simulink model "warplab_mimo_4x4"  (Simulink 6.5)
settings: Solver=ode45  StartTime=0.0  StopTime=20000  RelTol=1e-3
undefined symbols (not defined in the file): gcbh, xlBlockLoadCallback
libraries: xbsIndex_r4 x188
(part 2 of 17)

== system warplab_mimo_4x4/ System Generator ==
  2x System Clock : DiscretePulseGenerator  SampleTime=simulink_period
  Continuous Source : DiscretePulseGenerator  PulseType=Time based  Period=2*simulink_period  PulseWidth=50
  Terminator : Terminator
  Terminator1 : Terminator
  wires:
  2x System Clock/1 -> Terminator/1
  Continuous Source/1 -> Terminator1/1

== system warplab_mimo_4x4/CaptureDone ==
  In1 : Inport
  Inverter1 : S-Function  LoadFcn=xlBlockLoadCallback(gcbh);  FunctionName=sysgen  Parameters=ptable_  mask(Xilinx Inverter Block){infoedit=Bitwise logical negation (one's complement) operator., en_sgadvanced=, en=off, latency=0, dbl_ovrd_sgadvanced=, dbl_ovrd=off, xl_use_area_sgadvanced=, xl_use_area=off, xl_area=[0,0,0,0,0,0,0], has_advanced_control=0, sggui_pos=-1,-1,-1,-1, block_type=inv, block_version=8.2, sg_icon_stat=25,18,1,1,white,blue,0,1ab4a85f, sg_mask_display=|, sg_list_contents=, sg_blockgui_xml=}
      mask sg_mask_display=|
      | fprintf('','COMMENT: begin icon graphics');
      | patch([0 25 25 0 ],[0 0 18 18 ],[0.77 0.82 0.91]);
      | patch([8 5 9 5 8 13 14 15 20 16 12 9 13 9 12 16 20 15 14 13 8 ],[2 5 9 13 16 16 15 16 16 12 16 13 9 5 2 6 2 2 3 2 2 ],[0.98 0.96 0.92]);
      | plot([0 0 25 25 0 ],[0 18 18 0 0 ]);
      | fprintf('','COMMENT: end icon graphics');
      | fprintf('','COMMENT: begin icon text');
      | color('black');disp('not');
      | fprintf('','COMMENT: end icon text');
      mask prompts: infoedit ""; en_sgadvanced ""; en "Provide enable port"; dbl_ovrd_sgadvanced ""; dbl_ovrd "Override with doubles"; xl_use_area_sgadvanced ""; xl_use_area "Define FPGA area for resource estimation"; xl_area "FPGA area [slices, FFs, BRAMs, LUTs, IOBs, emb. mults, TBUFs]"; has_advanced_control ""; sggui_pos ""; block_type ""; block_version ""; sg_icon_stat ""; sg_mask_display ""; sg_list_contents ""; sg_blockgui_xml ""
      mask help: Bitwise logical negation (one's complement) operator.
      mask init: same as warplab_mimo_4x4/Inverter
      settings: CopyFcn=xlBlockMoveCallback(gcbh);  DeleteFcn=xlDestroyGui(gcbh);  ModelCloseFcn=xlDestroyGui(gcbh);  PreSaveFcn=xlBlockPreSaveCallback(gcbh);  PostSaveFcn=xlBlockPostSaveCallback(gcbh);  DestroyFcn=xlDestroyGui(gcbh);  OpenFcn=xlOpenGui(gcbh, 'inv_gui.xml', @xlmagicenablement, -1)  CloseFcn=xlDestroyGui(gcbh);  MoveFcn=xlBlockMoveCallback(gcbh);
      mask Help: eval('xlWeb(xlhtmldoclink(''Inverter''))');
      mask Display:
      | fprintf('','COMMENT: begin icon graphics');
      | patch([0 25 25 0 ],[0 0 18 18 ],[0.77 0.82 0.91]);
      | patch([8 5 9 5 8 13 14 15 20 16 12 9 13 9 12 16 20 15 14 13 8 ],[2 5 9 13 16 16 15 16 16 12 16 13 9 5 2 6 2 2 3 2 2 ],[0.98 0.96 0.92]);
      | plot([0 0 25 25 0 ],[0 18 18 0 0 ]);
      | fprintf('','COMMENT: end icon graphics');
      | fprintf('','COMMENT: begin icon text');
      | color('black');disp('not');
      | fprintf('','COMMENT: end icon text');
  zero3 : S-Function  LoadFcn=xlBlockLoadCallback(gcbh);  FunctionName=sysgen  Parameters=ptable_  mask(Xilinx Constant Block Block){arith_type_sgadvanced=, arith_type=Boolean, const=1, n_bits=1, bin_pt=0, explicit_period_sgadvanced=, explicit_period=off, period=1, dsp48_infoedit=The use of this block for DSP48 instructions is deprecated.  Please use the Opmode block., equ=P=C, opselect_sgadvanced=, opselect=C, inp2_sgadvanced=, inp2=PCIN>>17, opr_sgadvanced=, opr=+, inp1_sgadvanced=, inp1=P, carry_sgadvanced=, carry=CIN, dbl_ovrd_sgadvanced=, dbl_ovrd=off, has_advanced_control=0, sggui_pos=-1,-1,-1,-1, block_type=constant, block_version=VER_STRING_GOES_HERE, sg_icon_stat=20,18,0,1,white,blue,0,85613821, sg_mask_display=|, sg_list_contents=, sg_blockgui_xml=}
      mask sg_mask_display=|
      | fprintf('','COMMENT: begin icon graphics');
      | patch([0 55 55 0 ],[0 0 26 26 ],[0.77 0.82 0.91]);
      | patch([20 16 22 16 20 27 29 31 38 32 26 22 28 22 26 32 38 31 29 27 20 ],[3 7 13 19 23 23 21 23 23 17 23 19 13 7 3 9 3 3 5 3 3 ],[0.98 0.96 0.92]);
      | plot([0 0 55 55 0 ],[0 26 26 0 0 ]);
      | fprintf('','COMMENT: end icon graphics');
      | fprintf('','COMMENT: begin icon text');
      | color('black');port_label('output',1,'1');
      | fprintf('','COMMENT: end icon text');
      mask prompts: arith_type_sgadvanced ""; arith_type "Type"; const "Constant value"; n_bits "Number of bits"; bin_pt "Binary point"; explicit_period_sgadvanced ""; explicit_period "Sampled constant"; period "Sample period"; dsp48_infoedit ""; equ "DSP48 operation"; opselect_sgadvanced ""; opselect "Operation select"; inp2_sgadvanced ""; inp2 "Z mux"; opr_sgadvanced ""; opr "Operand"; inp1_sgadvanced ""; inp1 "YX muxes"; carry_sgadvanced ""; carry "Carry input"; dbl_ovrd_sgadvanced ""; dbl_ovrd "Override with doubles"; has_advanced_control ""; sggui_pos ""; block_type ""; block_version ""; sg_icon_stat ""; sg_mask_display ""; sg_list_contents ""; sg_blockgui_xml ""
      mask help: Xilinx Constant Block
      mask init:
      | try
      |   tmp_gcb = gcb;
      |   tmp_gcbh = gcbh;
      |   xlMungeMaskParams;
      |   block_config = 'sysgen_blockset:Constant_config';
      |   serialized_declarations = '{''arith_type''=>''Int'',''bin_pt''=>''Int'',''carry''=>''Int'',''const''=>''Double'',''dbl_ovrd''=>''Int'',''explicit_period''=>''Int'',''inp1''=>''Int'',''inp2''=>''Int'',''n_bits''=>''Int'',''opr''=>''Int'',''opselect''=>''Int'',''period''=>''Double''}';
      |   xlconstant_init();
      |   ptable_ = xlblockprep(get_param(tmp_gcb, 'MaskWSVariables'));
      | catch
      |   global dbgsysgen;
      |   if(~isempty(dbgsysgen) && dbgsysgen)
      |     e = regexprep(lasterr, '\n', '\nError: ');
      |     disp(['Error: While running MaskInit code on block ' tmp_gcb ': ' e]);
      |     error(e);
      |   end
      | end
      settings: CopyFcn=xlBlockMoveCallback(gcbh);  DeleteFcn=xlDestroyGui(gcbh);  ModelCloseFcn=xlDestroyGui(gcbh);  PreSaveFcn=xlBlockPreSaveCallback(gcbh);  PostSaveFcn=xlBlockPostSaveCallback(gcbh);  DestroyFcn=xlDestroyGui(gcbh);  OpenFcn=xlOpenGui(gcbh, 'constant_gui.xml', @constantenablement, @constantaction)  CloseFcn=xlDestroyGui(gcbh);  MoveFcn=xlBlockMoveCallback(gcbh);
      mask Help: eval('xlWeb(xlhtmldoclink(''Constant''))');
      mask StyleString: edit,popup(Boolean|Signed (2's comp)|Unsigned|DSP48 Instruction),edit,edit,edit,edit,checkbox,edit,edit,edit,edit,popup(C + A*B|PCIN + A*B|P + A*B|A * B|C + A:B|C - A:B|C|Custom),edit,popup(0|PCIN|P|C|PCIN>>17|P>>17),edit,popup(+|-),edit,popup(0|P|A:B|A*B|C|P+C|A:B+C),edit,popup(0|1|CIN|~SIGN(P or PCIN)|~SIGN(A*B or A:B)|~SIGND(A*B or A:B)),edit,checkbox,edit,edit,edit,edit,edit,edit,edit,edit
      mask Display:
      | fprintf('','COMMENT: begin icon graphics');
      | patch([0 55 55 0 ],[0 0 26 26 ],[0.77 0.82 0.91]);
      | patch([20 16 22 16 20 27 29 31 38 32 26 22 28 22 26 32 38 31 29 27 20 ],[3 7 13 19 23 23 21 23 23 17 23 19 13 7 3 9 3 3 5 3 3 ],[0.98 0.96 0.92]);
      | plot([0 0 55 55 0 ],[0 26 26 0 0 ]);
      | fprintf('','COMMENT: end icon graphics');
      | fprintf('','COMMENT: begin icon text');
      | color('black');port_label('output',1,'1');
      | fprintf('','COMMENT: end icon text');
  Out1_To_Register : Outport
  tag scope: en_out_13=global, out_13=global
  wires:
  In1/1 -> Inverter1/1
  Inverter1/1 -> [out_13]
  zero3/1 -> [en_out_13]

== system warplab_mimo_4x4/Mem_Control ==
  Start : Inport
  DoneReading : Inport  Port=2
  CaptOffset : Inport  Port=3
  AddSub1 : S-Function  LoadFcn=xlBlockLoadCallback(gcbh);  FunctionName=sysgen  Parameters=ptable_  mask(Xilinx Adder/Subtractor Block){mode_sgadvanced=, mode=Subtraction, use_carryin_sgadvanced=, use_carryin=off, use_carryout_sgadvanced=, use_carryout=off, en_sgadvanced=, en=off, latency=0, precision_sgadvanced=, precision=User Defined, arith_type_sgadvanced=, arith_type=Unsigned, n_bits=14, bin_pt=0, quantization_sgadvanced=, quantization=Truncate, overflow_sgadvanced=, overflow=Wrap, dbl_ovrd_sgadvanced=, dbl_ovrd=off, use_behavioral_HDL_sgadvanced=, use_behavioral_HDL=off, pipelined_sgadvanced=, pipelined=off, use_rpm_sgadvanced=, use_rpm=on, xl_use_area_sgadvanced=, xl_use_area=off, xl_area=[0,0,0,0,0,0,0], has_advanced_control=0, sggui_pos=-1,-1,-1,-1, block_type=addsub, block_version=8.2, sg_icon_stat=45,38,2,1,white,blue,0,f28631c4, sg_mask_display=|, sg_list_contents=, sg_blockgui_xml=}
      mask sg_mask_display=|
      | fprintf('','COMMENT: begin icon graphics');
      | patch([0 45 45 0 ],[0 0 38 38 ],[0.77 0.82 0.91]);
      | patch([12 6 15 6 12 22 25 28 39 31 23 17 26 17 23 31 39 28 25 22 12 ],[4 10 19 28 34 34 31 34 34 26 34 28 19 10 4 12 4 4 7 4 4 ],[0.98 0.96 0.92]);
      | plot([0 0 45 45 0 ],[0 38 38 0 0 ]);
      | fprintf('','COMMENT: end icon graphics');
      | fprintf('','COMMENT: begin icon text');
      | color('black');port_label('input',1,'a');
      | color('black');port_label('input',2,'b');
      | color('black');port_label('output',1,'\bf{a - b}','texmode','on');
      | fprintf('','COMMENT: end icon text');
      mask prompts: mode_sgadvanced ""; mode "Operation"; use_carryin_sgadvanced ""; use_carryin "Provide carry-in port"; use_carryout_sgadvanced ""; use_carryout "Provide carry-out port"; en_sgadvanced ""; en "Provide enable port"; precision_sgadvanced ""; arith_type_sgadvanced ""; arith_type "Output type"; n_bits "Number of bits"; bin_pt "Binary point"; quantization_sgadvanced ""; overflow_sgadvanced ""; dbl_ovrd_sgadvanced ""; dbl_ovrd "Override with doubles"; use_behavioral_HDL_sgadvanced ""; use_behavioral_HDL "Use behavioral HDL (otherwise use core)"; pipelined_sgadvanced ""; pipelined "Pipeline for maximum performance"; use_rpm_sgadvanced ""; use_rpm "Use core placement information"; xl_use_area_sgadvanced ""; xl_use_area "Define FPGA area for resource estimation"; xl_area "FPGA area [slices, FFs, BRAMs, LUTs, IOBs, emb. mults, TBUFs]"; has_advanced_control ""; sggui_pos ""; block_type ""; block_version ""; sg_icon_stat ""; sg_mask_display ""; sg_list_contents ""; sg_blockgui_xml ""
      mask help: Xilinx Adder/Subtractor
      mask init:
      | try
      |   tmp_gcb = gcb;
      |   tmp_gcbh = gcbh;
      |   xlMungeMaskParams;
      |   block_config = 'sysgen_blockset:Addsub_config';
      |   serialized_declarations = '{''arith_type''=>''Int'',''bin_pt''=>''Int'',''en''=>''Int'',''latency''=>''Int'',''mode''=>''Int'',''n_bits''=>''Int'',''overflow''=>''Int'',''pipelined''=>''Int'',''precision''=>''Int'',''quantization''=>''Int'',''rst''=>''Int'',''use_behavioral_HDL''=>''Int'',''use_carryin''=>''Int'',''use_carryout''=>''Int'',''use_rpm''=>''Int''}';
      |   ptable_ = xlblockprep(get_param(tmp_gcb, 'MaskWSVariables'));
      | catch
      |   global dbgsysgen;
      |   if(~isempty(dbgsysgen) && dbgsysgen)
      |     e = regexprep(lasterr, '\n', '\nError: ');
      |     disp(['Error: While running MaskInit code on block ' tmp_gcb ': ' e]);
      |     error(e);
      |   end
      | end
      settings: CopyFcn=xlBlockMoveCallback(gcbh);  DeleteFcn=xlDestroyGui(gcbh);  ModelCloseFcn=xlDestroyGui(gcbh);  PreSaveFcn=xlBlockPreSaveCallback(gcbh);  PostSaveFcn=xlBlockPostSaveCallback(gcbh);  DestroyFcn=xlDestroyGui(gcbh);  OpenFcn=xlOpenGui(gcbh, 'addsub_gui.xml', @addsubenablement, -1)  CloseFcn=xlDestroyGui(gcbh);  MoveFcn=xlBlockMoveCallback(gcbh);
      mask Help: eval('xlWeb(xlhtmldoclink(''AddSub''))');
      mask StyleString: edit,popup(Addition|Subtraction|Addition or Subtraction),edit,checkbox,edit,checkbox,edit,checkbox,edit,edit,popup(Full|User Defined),edit,popup(Signed  (2's comp)|Unsigned),edit,edit,edit,popup(Truncate|Round  (unbiased: +/- Inf)),edit,popup(Wrap|Saturate|Flag as error),edit,checkbox,edit,checkbox,edit,checkbox,edit,checkbox,edit,checkbox,edit,edit,edit,edit,edit,edit,edit,edit,edit
      mask Display:
      | fprintf('','COMMENT: begin icon graphics');
      | patch([0 45 45 0 ],[0 0 38 38 ],[0.77 0.82 0.91]);
      | patch([12 6 15 6 12 22 25 28 39 31 23 17 26 17 23 31 39 28 25 22 12 ],[4 10 19 28 34 34 31 34 34 26 34 28 19 10 4 12 4 4 7 4 4 ],[0.98 0.96 0.92]);
      | plot([0 0 45 45 0 ],[0 38 38 0 0 ]);
      | fprintf('','COMMENT: end icon graphics');
      | fprintf('','COMMENT: begin icon text');
      | color('black');port_label('input',1,'a');
      | color('black');port_label('input',2,'b');
      | color('black');port_label('output',1,'\bf{a - b}','texmode','on');
      | fprintf('','COMMENT: end icon text');
  Convert1 : S-Function  LoadFcn=xlBlockLoadCallback(gcbh);  FunctionName=sysgen  Parameters=ptable_  mask(Xilinx Type Converter Block){infoedit=Hardware notes: rounding and saturating require hardware resources; truncating and wrapping do not., arith_type_sgadvanced=, arith_type=Boolean, n_bits=16, bin_pt=14, quantization_sgadvanced=, quantization=Truncate, overflow_sgadvanced=, overflow=Wrap, latency=0, dbl_ovrd_sgadvanced=, dbl_ovrd=off, pipeline_sgadvanced=, pipeline=off, xl_use_area_sgadvanced=, xl_use_area=off, xl_area=[0,0,0,0,0,0,0], has_advanced_control=0, sggui_pos=20,20,374,375, block_type=convert, block_version=8.2, sg_icon_stat=35,18,1,1,white,blue,0,0eb6e735, sg_mask_display=|, sg_list_contents=, sg_blockgui_xml=}
      mask sg_mask_display=|
      | fprintf('','COMMENT: begin icon graphics');
      | patch([0 35 35 0 ],[0 0 18 18 ],[0.77 0.82 0.91]);
      | patch([13 10 14 10 13 18 19 20 25 21 17 14 18 14 17 21 25 20 19 18 13 ],[2 5 9 13 16 16 15 16 16 12 16 13 9 5 2 6 2 2 3 2 2 ],[0.98 0.96 0.92]);
      | plot([0 0 35 35 0 ],[0 18 18 0 0 ]);
      | fprintf('','COMMENT: end icon graphics');
      | fprintf('','COMMENT: begin icon text');
      | color('black');port_label('output',1,'cast');
      | fprintf('','COMMENT: end icon text');
      mask prompts: infoedit ""; arith_type_sgadvanced ""; arith_type "Type"; n_bits "Number of bits"; bin_pt "Binary point"; quantization_sgadvanced ""; overflow_sgadvanced ""; dbl_ovrd_sgadvanced ""; dbl_ovrd "Override with doubles"; pipeline_sgadvanced ""; pipeline "Pipeline for maximum performance"; xl_use_area_sgadvanced ""; xl_use_area "Define FPGA area for resource estimation"; xl_area "FPGA area [slices, FFs, BRAMs, LUTs, IOBs, emb. mults, TBUFs]"; has_advanced_control ""; sggui_pos ""; block_type ""; block_version ""; sg_icon_stat ""; sg_mask_display ""; sg_list_contents ""; sg_blockgui_xml ""
      mask help: Hardware notes: rounding and saturating require hardware resources; truncating and wrapping do not.
      mask init:
      | try
      |   tmp_gcb = gcb;
      |   tmp_gcbh = gcbh;
      |   xlMungeMaskParams;
      |   block_config = 'sysgen_blockset:Convert_config';
      |   serialized_declarations = '{''arith_type''=>''Int'',''bin_pt''=>''Int'',''latency''=>''Int'',''n_bits''=>''Int'',''overflow''=>''Int'',''pipeline''=>''Int'',''quantization''=>''Int'',''sim_engine''=>''Int'',''sysgen_root''=>''String''}';
      |   xlconvert_init();
      |   ptable_ = xlblockprep(get_param(tmp_gcb, 'MaskWSVariables'));
      | catch
      |   global dbgsysgen;
      |   if(~isempty(dbgsysgen) && dbgsysgen)
      |     e = regexprep(lasterr, '\n', '\nError: ');
      |     disp(['Error: While running MaskInit code on block ' tmp_gcb ': ' e]);
      |     error(e);
      |   end
      | end
      settings: CopyFcn=xlBlockMoveCallback(gcbh);  DeleteFcn=xlDestroyGui(gcbh);  ModelCloseFcn=xlDestroyGui(gcbh);  PreSaveFcn=xlBlockPreSaveCallback(gcbh);  PostSaveFcn=xlBlockPostSaveCallback(gcbh);  DestroyFcn=xlDestroyGui(gcbh);  OpenFcn=xlOpenGui(gcbh, 'convert_gui.xml', @convertenablement, -1)  CloseFcn=xlDestroyGui(gcbh);  MoveFcn=xlBlockMoveCallback(gcbh);
      mask Help: eval('xlWeb(xlhtmldoclink(''Convert''))');
      mask StyleString: edit,edit,popup(Boolean|Signed  (2's comp)|Unsigned),edit,edit,edit,popup(Truncate|Round  (unbiased: +/- Inf)|Round  (unbiased: Even Values)),edit,popup(Wrap|Saturate|Flag as error),edit,edit,checkbox,edit,checkbox,edit,checkbox,edit,edit,edit,edit,edit,edit,edit,edit,edit
      mask Display:
      | fprintf('','COMMENT: begin icon graphics');
      | patch([0 35 35 0 ],[0 0 18 18 ],[0.77 0.82 0.91]);
      | patch([13 10 14 10 13 18 19 20 25 21 17 14 18 14 17 21 25 20 19 18 13 ],[2 5 9 13 16 16 15 16 16 12 16 13 9 5 2 6 2 2 3 2 2 ],[0.98 0.96 0.92]);
      | plot([0 0 35 35 0 ],[0 18 18 0 0 ]);
      | fprintf('','COMMENT: end icon graphics');
      | fprintf('','COMMENT: begin icon text');
      | color('black');port_label('output',1,'cast');
      | fprintf('','COMMENT: end icon text');
  Delay : S-Function  LoadFcn=xlBlockLoadCallback(gcbh);  FunctionName=sysgen  Parameters=ptable_  mask(Xilinx Delay Block){infoedit=Hardware notes: A delay line is a chain, each link of which is an SRL16 followed by a flip-flop. If register retiming is enabled, the delay line is a chain of flip-flops., en_sgadvanced=, en=off, latency=1, dbl_ovrd_sgadvanced=, dbl_ovrd=off, reg_retiming_sgadvanced=, reg_retiming=off, xl_use_area_sgadvanced=, xl_use_area=off, xl_area=[0,0,0,0,0,0,0], has_advanced_control=0, sggui_pos=-1,-1,-1,-1, block_type=delay, block_version=8.2, sg_icon_stat=30,30,1,1,white,blue,0,fc531c0e, sg_mask_display=|, sg_list_contents=, sg_blockgui_xml=}
      mask sg_mask_display=|
      | fprintf('','COMMENT: begin icon graphics');
      | patch([0 30 30 0 ],[0 0 30 30 ],[0.77 0.82 0.91]);
      | patch([7 2 9 2 7 15 17 19 27 20 14 9 15 9 14 20 27 19 17 15 7 ],[3 8 15 22 27 27 25 27 27 20 26 21 15 9 4 10 3 3 5 3 3 ],[0.98 0.96 0.92]);
      | plot([0 0 30 30 0 ],[0 30 30 0 0 ]);
      | fprintf('','COMMENT: end icon graphics');
      | fprintf('','COMMENT: begin icon text');
      | color('black');disp('z^{-1}','texmode','on');
      | fprintf('','COMMENT: end icon text');
      mask prompts: infoedit ""; en_sgadvanced ""; en "Provide enable port"; dbl_ovrd_sgadvanced ""; dbl_ovrd "Override with doubles"; reg_retiming_sgadvanced ""; reg_retiming "Implement using behavioral HDL."; xl_use_area_sgadvanced ""; xl_use_area "Define FPGA area for resource estimation"; xl_area "FPGA area [slices, FFs, BRAMs, LUTs, IOBs, emb. mults, TBUFs]"; has_advanced_control ""; sggui_pos ""; block_type ""; block_version ""; sg_icon_stat ""; sg_mask_display ""; sg_list_contents ""; sg_blockgui_xml ""
      mask help: Hardware notes: A delay line is a chain, each link of which is an SRL16 followed by a flip-flop.
      mask init:
      | try
      |   tmp_gcb = gcb;
      |   tmp_gcbh = gcbh;
      |   xlMungeMaskParams;
      |   block_config = 'sysgen_blockset:Delay_config';
      |   serialized_declarations = '{''dbl_ovrd''=>''Int'',''en''=>''Int'',''latency''=>''Int'',''reg_retiming''=>''Int''}';
      |   ptable_ = xlblockprep(get_param(tmp_gcb, 'MaskWSVariables'));
      | catch
      |   global dbgsysgen;
      |   if(~isempty(dbgsysgen) && dbgsysgen)
      |     e = regexprep(lasterr, '\n', '\nError: ');
      |     disp(['Error: While running MaskInit code on block ' tmp_gcb ': ' e]);
      |     error(e);
      |   end
      | end
      settings: CopyFcn=xlBlockMoveCallback(gcbh);  DeleteFcn=xlDestroyGui(gcbh);  ModelCloseFcn=xlDestroyGui(gcbh);  PreSaveFcn=xlBlockPreSaveCallback(gcbh);  PostSaveFcn=xlBlockPostSaveCallback(gcbh);  DestroyFcn=xlDestroyGui(gcbh);  OpenFcn=xlOpenGui(gcbh, 'delay_gui.xml', @xlmagicenablement, -1)  CloseFcn=xlDestroyGui(gcbh);  MoveFcn=xlBlockMoveCallback(gcbh);
      mask Help: eval('xlWeb(xlhtmldoclink(''Delay''))');
      mask Display:
      | fprintf('','COMMENT: begin icon graphics');
      | patch([0 30 30 0 ],[0 0 30 30 ],[0.77 0.82 0.91]);
      | patch([7 2 9 2 7 15 17 19 27 20 14 9 15 9 14 20 27 19 17 15 7 ],[3 8 15 22 27 27 25 27 27 20 26 21 15 9 4 10 3 3 5 3 3 ],[0.98 0.96 0.92]);
      | plot([0 0 30 30 0 ],[0 30 30 0 0 ]);
      | fprintf('','COMMENT: end icon graphics');
      | fprintf('','COMMENT: begin icon text');
      | color('black');disp('z^{-1}','texmode','on');
      | fprintf('','COMMENT: end icon text');
  Logical : S-Function  LoadFcn=xlBlockLoadCallback(gcbh);  FunctionName=sysgen  Parameters=ptable_  mask(Xilinx Logical Block Block){logical_function_sgadvanced=, logical_function=AND, inputs=2, en_sgadvanced=, en=off, latency=0, precision_sgadvanced=, precision=Full, arith_type_sgadvanced=, arith_type=Unsigned, n_bits=16, bin_pt=0, align_bp_sgadvanced=, align_bp=on, dbl_ovrd_sgadvanced=, dbl_ovrd=off, xl_use_area_sgadvanced=, xl_use_area=off, xl_area=[0,0,0,0,0,0,0], overflow=, quantization=, has_advanced_control=0, sggui_pos=-1,-1,-1,-1, block_type=logical, block_version=8.2, sg_icon_stat=35,42,2,1,white,blue,0,087b5522, sg_mask_display=|, sg_list_contents=, sg_blockgui_xml=}
      mask sg_mask_display=|
      | fprintf('','COMMENT: begin icon graphics');
      | patch([0 35 35 0 ],[0 0 42 42 ],[0.77 0.82 0.91]);
      | patch([8 2 10 2 8 17 20 23 33 25 18 13 21 13 18 25 33 23 20 17 8 ],[7 13 21 29 35 35 32 35 35 27 34 29 21 13 8 15 7 7 10 7 7 ],[0.98 0.96 0.92]);
      | plot([0 0 35 35 0 ],[0 42 42 0 0 ]);
      | fprintf('','COMMENT: end icon graphics');
      | fprintf('','COMMENT: begin icon text');
      | color('black');disp('\newlineand\newlinez^{-0}','texmode','on');
      | fprintf('','COMMENT: end icon text');
      mask prompts: logical_function_sgadvanced ""; logical_function "Logical function"; inputs "Number of inputs"; en_sgadvanced ""; en "Provide enable port"; precision_sgadvanced ""; arith_type_sgadvanced ""; arith_type "Output Type"; n_bits "Number of bits"; bin_pt "Binary point"; align_bp_sgadvanced ""; align_bp "Align binary point"; dbl_ovrd_sgadvanced ""; dbl_ovrd "Override with doubles"; xl_use_area_sgadvanced ""; xl_use_area "Define FPGA area for resource estimation"; xl_area "FPGA area [slices, FFs, BRAMs, LUTs, IOBs, emb. mults, TBUFs]"; overflow ""; quantization ""; has_advanced_control ""; sggui_pos ""; block_type ""; block_version ""; sg_icon_stat ""; sg_mask_display ""; sg_list_contents ""; sg_blockgui_xml ""
      mask help: Xilinx Logical Block
      mask init: same as warplab_mimo_4x4/Logical
      settings: CopyFcn=xlBlockMoveCallback(gcbh);  DeleteFcn=xlDestroyGui(gcbh);  ModelCloseFcn=xlDestroyGui(gcbh);  PreSaveFcn=xlBlockPreSaveCallback(gcbh);  PostSaveFcn=xlBlockPostSaveCallback(gcbh);  DestroyFcn=xlDestroyGui(gcbh);  OpenFcn=xlOpenGui(gcbh, 'logical_gui.xml', @logicalenablement, -1)  CloseFcn=xlDestroyGui(gcbh);  MoveFcn=xlBlockMoveCallback(gcbh);
      mask Help: eval('xlWeb(xlhtmldoclink(''Logical''))');
      mask StyleString: edit,popup(AND|NAND|OR|NOR|XOR|XNOR),edit,edit,checkbox,edit,edit,popup(Full|User Defined),edit,popup(Signed  (2's comp)|Unsigned),edit,edit,edit,checkbox,edit,checkbox,edit,checkbox,edit,edit,edit,edit,edit,edit,edit,edit,edit,edit,edit
      mask Display:
      | fprintf('','COMMENT: begin icon graphics');
      | patch([0 35 35 0 ],[0 0 42 42 ],[0.77 0.82 0.91]);
      | patch([8 2 10 2 8 17 20 23 33 25 18 13 21 13 18 25 33 23 20 17 8 ],[7 13 21 29 35 35 32 35 35 27 34 29 21 13 8 15 7 7 10 7 7 ],[0.98 0.96 0.92]);
      | plot([0 0 35 35 0 ],[0 42 42 0 0 ]);
      | fprintf('','COMMENT: end icon graphics');
      | fprintf('','COMMENT: begin icon text');
      | color('black');disp('\newlineand\newlinez^{-0}','texmode','on');
      | fprintf('','COMMENT: end icon text');
  Logical2 : S-Function  LoadFcn=xlBlockLoadCallback(gcbh);  FunctionName=sysgen  Parameters=ptable_  mask(Xilinx Logical Block Block){logical_function_sgadvanced=, logical_function=AND, inputs=2, en_sgadvanced=, en=off, latency=0, precision_sgadvanced=, precision=Full, arith_type_sgadvanced=, arith_type=Unsigned, n_bits=16, bin_pt=0, align_bp_sgadvanced=, align_bp=on, dbl_ovrd_sgadvanced=, dbl_ovrd=off, xl_use_area_sgadvanced=, xl_use_area=off, xl_area=[0,0,0,0,0,0,0], overflow=, quantization=, has_advanced_control=0, sggui_pos=-1,-1,-1,-1, block_type=logical, block_version=8.2, sg_icon_stat=35,42,2,1,white,blue,0,087b5522, sg_mask_display=|, sg_list_contents=, sg_blockgui_xml=}
      mask sg_mask_display=|
      | fprintf('','COMMENT: begin icon graphics');
      | patch([0 35 35 0 ],[0 0 42 42 ],[0.77 0.82 0.91]);
      | patch([8 2 10 2 8 17 20 23 33 25 18 13 21 13 18 25 33 23 20 17 8 ],[7 13 21 29 35 35 32 35 35 27 34 29 21 13 8 15 7 7 10 7 7 ],[0.98 0.96 0.92]);
      | plot([0 0 35 35 0 ],[0 42 42 0 0 ]);
      | fprintf('','COMMENT: end icon graphics');
      | fprintf('','COMMENT: begin icon text');
      | color('black');disp('\newlineand\newlinez^{-0}','texmode','on');
      | fprintf('','COMMENT: end icon text');
      mask prompts: logical_function_sgadvanced ""; logical_function "Logical function"; inputs "Number of inputs"; en_sgadvanced ""; en "Provide enable port"; precision_sgadvanced ""; arith_type_sgadvanced ""; arith_type "Output Type"; n_bits "Number of bits"; bin_pt "Binary point"; align_bp_sgadvanced ""; align_bp "Align binary point"; dbl_ovrd_sgadvanced ""; dbl_ovrd "Override with doubles"; xl_use_area_sgadvanced ""; xl_use_area "Define FPGA area for resource estimation"; xl_area "FPGA area [slices, FFs, BRAMs, LUTs, IOBs, emb. mults, TBUFs]"; overflow ""; quantization ""; has_advanced_control ""; sggui_pos ""; block_type ""; block_version ""; sg_icon_stat ""; sg_mask_display ""; sg_list_contents ""; sg_blockgui_xml ""
      mask help: Xilinx Logical Block
      mask init: same as warplab_mimo_4x4/Logical
      settings: CopyFcn=xlBlockMoveCallback(gcbh);  DeleteFcn=xlDestroyGui(gcbh);  ModelCloseFcn=xlDestroyGui(gcbh);  PreSaveFcn=xlBlockPreSaveCallback(gcbh);  PostSaveFcn=xlBlockPostSaveCallback(gcbh);  DestroyFcn=xlDestroyGui(gcbh);  OpenFcn=xlOpenGui(gcbh, 'logical_gui.xml', @logicalenablement, -1)  CloseFcn=xlDestroyGui(gcbh);  MoveFcn=xlBlockMoveCallback(gcbh);
      mask Help: eval('xlWeb(xlhtmldoclink(''Logical''))');
      mask StyleString: edit,popup(AND|NAND|OR|NOR|XOR|XNOR),edit,edit,checkbox,edit,edit,popup(Full|User Defined),edit,popup(Signed  (2's comp)|Unsigned),edit,edit,edit,checkbox,edit,checkbox,edit,checkbox,edit,edit,edit,edit,edit,edit,edit,edit,edit,edit,edit
      mask Display:
      | fprintf('','COMMENT: begin icon graphics');
      | patch([0 35 35 0 ],[0 0 42 42 ],[0.77 0.82 0.91]);
      | patch([8 2 10 2 8 17 20 23 33 25 18 13 21 13 18 25 33 23 20 17 8 ],[7 13 21 29 35 35 32 35 35 27 34 29 21 13 8 15 7 7 10 7 7 ],[0.98 0.96 0.92]);
      | plot([0 0 35 35 0 ],[0 42 42 0 0 ]);
      | fprintf('','COMMENT: end icon graphics');
      | fprintf('','COMMENT: begin icon text');
      | color('black');disp('\newlineand\newlinez^{-0}','texmode','on');
      | fprintf('','COMMENT: end icon text');
  Register : S-Function  LoadFcn=xlBlockLoadCallback(gcbh);  FunctionName=sysgen  Parameters=ptable_  mask(Xilinx Register Block){init=0, rst_sgadvanced=, rst=off, en_sgadvanced=, en=on, dbl_ovrd_sgadvanced=, dbl_ovrd=off, xl_use_area_sgadvanced=, xl_use_area=off, xl_area=[0,0,0,0,0,0,0], has_advanced_control=0, sggui_pos=-1,-1,-1,-1, block_type=register, block_version=8.2, sg_icon_stat=50,40,2,1,white,blue,0,cc3303a0, sg_mask_display=|, sg_list_contents=, sg_blockgui_xml=}
      mask sg_mask_display=|
      | fprintf('','COMMENT: begin icon graphics');
      | patch([0 50 50 0 ],[0 0 40 40 ],[0.77 0.82 0.91]);
      | patch([15 8 17 8 15 26 29 32 43 34 25 19 29 19 25 34 43 32 29 26 15 ],[4 11 20 29 36 36 33 36 36 27 36 30 20 10 4 13 4 4 7 4 4 ],[0.98 0.96 0.92]);
      | plot([0 0 50 50 0 ],[0 40 40 0 0 ]);
      | fprintf('','COMMENT: end icon graphics');
      | fprintf('','COMMENT: begin icon text');
      | color('black');port_label('input',1,'d');
      | color('black');port_label('input',2,'en');
      | color('black');port_label('output',1,'q');
      | color('black');disp('\bf{z^{-1}}','texmode','on');
      | fprintf('','COMMENT: end icon text');
      mask prompts: init "Initial value"; rst_sgadvanced ""; rst "Provide synchronous reset port"; en_sgadvanced ""; en "Provide enable port"; dbl_ovrd_sgadvanced ""; dbl_ovrd "Override with doubles"; xl_use_area_sgadvanced ""; xl_use_area "Define FPGA area for resource estimation"; xl_area "FPGA area [slices, FFs, BRAMs, LUTs, IOBs, emb. mults, TBUFs]"; has_advanced_control ""; sggui_pos ""; block_type ""; block_version ""; sg_icon_stat ""; sg_mask_display ""; sg_list_contents ""; sg_blockgui_xml ""
      mask help: Xilinx Register
      mask init:
      | try
      |   tmp_gcb = gcb;
      |   tmp_gcbh = gcbh;
      |   xlMungeMaskParams;
      |   block_config = 'sysgen_blockset:Register_config';
      |   serialized_declarations = '{''dbl_ovrd''=>''Int'',''en''=>''Int'',''init''=>''Double'',''rst''=>''Int''}';
      |   xlregister_init();
      |   ptable_ = xlblockprep(get_param(tmp_gcb, 'MaskWSVariables'));
      | catch
      |   global dbgsysgen;
      |   if(~isempty(dbgsysgen) && dbgsysgen)
      |     e = regexprep(lasterr, '\n', '\nError: ');
      |     disp(['Error: While running MaskInit code on block ' tmp_gcb ': ' e]);
      |     error(e);
      |   end
      | end
      settings: CopyFcn=xlBlockMoveCallback(gcbh);  DeleteFcn=xlDestroyGui(gcbh);  ModelCloseFcn=xlDestroyGui(gcbh);  PreSaveFcn=xlBlockPreSaveCallback(gcbh);  PostSaveFcn=xlBlockPostSaveCallback(gcbh);  DestroyFcn=xlDestroyGui(gcbh);  OpenFcn=xlOpenGui(gcbh, 'register_gui.xml', @xlmagicenablement, -1)  CloseFcn=xlDestroyGui(gcbh);  MoveFcn=xlBlockMoveCallback(gcbh);
      mask Help: eval('xlWeb(xlhtmldoclink(''Register''))');
      mask Display:
      | fprintf('','COMMENT: begin icon graphics');
      | patch([0 50 50 0 ],[0 0 40 40 ],[0.77 0.82 0.91]);
      | patch([15 8 17 8 15 26 29 32 43 34 25 19 29 19 25 34 43 32 29 26 15 ],[4 11 20 29 36 36 33 36 36 27 36 30 20 10 4 13 4 4 7 4 4 ],[0.98 0.96 0.92]);
      | plot([0 0 50 50 0 ],[0 40 40 0 0 ]);
      | fprintf('','COMMENT: end icon graphics');
      | fprintf('','COMMENT: begin icon text');
      | color('black');port_label('input',1,'d');
      | color('black');port_label('input',2,'en');
      | color('black');port_label('output',1,'q');
      | color('black');disp('\bf{z^{-1}}','texmode','on');
      | fprintf('','COMMENT: end icon text');
  Relational : S-Function  LoadFcn=xlBlockLoadCallback(gcbh);  FunctionName=sysgen  Parameters=ptable_  mask(Xilinx Arithmetic Relational Operator Block){mode_sgadvanced=, mode=a=b, en_sgadvanced=, en=off, latency=0, dbl_ovrd_sgadvanced=, dbl_ovrd=off, xl_use_area_sgadvanced=, xl_use_area=off, xl_area=[0,0,0,0,0,0,0], has_advanced_control=0, sggui_pos=-1,-1,-1,-1, block_type=relational, block_version=8.2, sg_icon_stat=45,84,2,1,white,blue,0,1b68ef8e, sg_mask_display=|, sg_list_contents=, sg_blockgui_xml=}
      mask sg_mask_display=|
      | fprintf('','COMMENT: begin icon graphics');
      | patch([0 45 45 0 ],[0 0 84 84 ],[0.77 0.82 0.91]);
      | patch([10 3 14 3 10 22 25 28 41 31 21 14 25 14 21 31 41 28 25 22 10 ],[24 31 42 53 60 60 57 60 60 50 60 53 42 31 24 34 24 24 27 24 24 ],[0.98 0.96 0.92]);
      | plot([0 0 45 45 0 ],[0 84 84 0 0 ]);
      | fprintf('','COMMENT: end icon graphics');
      | fprintf('','COMMENT: begin icon text');
      | color('black');port_label('input',1,'a');
      | color('black');port_label('input',2,'b');
      | color('black');disp('\newline\bf{a=b}\newlinez^{-0}','texmode','on');
      | fprintf('','COMMENT: end icon text');
      mask prompts: mode_sgadvanced ""; mode "Comparison:"; en_sgadvanced ""; en "Provide enable port"; dbl_ovrd_sgadvanced ""; dbl_ovrd "Override with doubles"; xl_use_area_sgadvanced ""; xl_use_area "Define FPGA area for resource estimation"; xl_area "FPGA area [slices, FFs, BRAMs, LUTs, IOBs, emb. mults, TBUFs]"; has_advanced_control ""; sggui_pos ""; block_type ""; block_version ""; sg_icon_stat ""; sg_mask_display ""; sg_list_contents ""; sg_blockgui_xml ""
      mask help: Xilinx Arithmetic Relational Operator
      mask init: same as warplab_mimo_4x4/Relational
      settings: CopyFcn=xlBlockMoveCallback(gcbh);  DeleteFcn=xlDestroyGui(gcbh);  ModelCloseFcn=xlDestroyGui(gcbh);  PreSaveFcn=xlBlockPreSaveCallback(gcbh);  PostSaveFcn=xlBlockPostSaveCallback(gcbh);  DestroyFcn=xlDestroyGui(gcbh);  OpenFcn=xlOpenGui(gcbh, 'relational_gui.xml', @xlmagicenablement, -1)  CloseFcn=xlDestroyGui(gcbh);  MoveFcn=xlBlockMoveCallback(gcbh);
      mask Help: eval('xlWeb(xlhtmldoclink(''Relational''))');
      mask StyleString: edit,popup(a=b|a!=b|a<b|a>b|a<=b|a>=b),edit,checkbox,edit,edit,checkbox,edit,checkbox,edit,edit,edit,edit,edit,edit,edit,edit,edit
      mask Display:
      | fprintf('','COMMENT: begin icon graphics');
      | patch([0 45 45 0 ],[0 0 84 84 ],[0.77 0.82 0.91]);
      | patch([10 3 14 3 10 22 25 28 41 31 21 14 25 14 21 31 41 28 25 22 10 ],[24 31 42 53 60 60 57 60 60 50 60 53 42 31 24 34 24 24 27 24 24 ],[0.98 0.96 0.92]);
      | plot([0 0 45 45 0 ],[0 84 84 0 0 ]);
      | fprintf('','COMMENT: end icon graphics');
      | fprintf('','COMMENT: begin icon text');
      | color('black');port_label('input',1,'a');
      | color('black');port_label('input',2,'b');
      | color('black');disp('\newline\bf{a=b}\newlinez^{-0}','texmode','on');
      | fprintf('','COMMENT: end icon text');
  Rx Addr Counter : S-Function  LoadFcn=xlBlockLoadCallback(gcbh);  FunctionName=sysgen  Parameters=ptable_  mask(Xilinx Counter Block){infoedit=Hardware notes: Free running counters are the least expensive in hardware.  A count limited counter is implemented by combining a counter with a comparator., cnt_type_sgadvanced=, cnt_type=Free Running, cnt_to=Inf, operation_sgadvanced=, operation=Up, start_count=0, cnt_by_val=1, arith_type_sgadvanced=, arith_type=Unsigned, n_bits=14, bin_pt=0, load_pin_sgadvanced=, load_pin=off, rst_sgadvanced=, rst=off, en_sgadvanced=, en=off, explicit_period_sgadvanced=, explicit_period=on, period=1, dbl_ovrd_sgadvanced=, dbl_ovrd=off, use_behavioral_HDL_sgadvanced=, use_behavioral_HDL=off, use_rpm_sgadvanced=, use_rpm=off, xl_use_area_sgadvanced=, xl_use_area=off, xl_area=[0,0,0,0,0,0,0], xlcconfig=, has_advanced_control=0, sggui_pos=20,20,356,630, block_type=counter, block_version=8.2, sg_icon_stat=50,30,0,1,white,blue,0,115399eb, sg_mask_display=|, sg_list_contents=, sg_blockgui_xml=}
      mask sg_mask_display=|
      | fprintf('','COMMENT: begin icon graphics');
      | patch([0 50 50 0 ],[0 0 30 30 ],[0.77 0.82 0.91]);
      | patch([17 12 19 12 17 25 27 29 37 30 24 19 25 19 24 30 37 29 27 25 17 ],[3 8 15 22 27 27 25 27 27 20 26 21 15 9 4 10 3 3 5 3 3 ],[0.98 0.96 0.92]);
      | plot([0 0 50 50 0 ],[0 30 30 0 0 ]);
      | fprintf('','COMMENT: end icon graphics');
      | fprintf('','COMMENT: begin icon text');
      | color('black');port_label('output',1,'out');
      | fprintf('','COMMENT: end icon text');
      mask prompts: infoedit ""; cnt_type_sgadvanced ""; cnt_type "Counter type"; cnt_to "Count to value"; operation_sgadvanced ""; operation "Count direction"; start_count "Initial value"; cnt_by_val "Step"; arith_type_sgadvanced ""; arith_type "Output type"; n_bits "Number of bits"; bin_pt "Binary point"; load_pin_sgadvanced ""; load_pin "Provide load port"; rst_sgadvanced ""; rst "Provide synchronous reset port"; en_sgadvanced ""; en "Provide enable port"; explicit_period_sgadvanced ""; explicit_period "Sample period source"; period "Explicit period"; dbl_ovrd_sgadvanced ""; dbl_ovrd "Override with doubles"; use_behavioral_HDL_sgadvanced ""; use_behavioral_HDL "Use behavioral HDL (otherwise use core)"; use_rpm_sgadvanced ""; use_rpm "Use pre-defined core placement information"; xl_use_area_sgadvanced ""; xl_use_area "Define FPGA area for resource estimation"; xl_area "FPGA area [slices, FFs, BRAMs, LUTs, IOBs, emb. mults, TBUFs]"; xlcconfig ""; has_advanced_control ""; sggui_pos ""; block_type ""; block_version ""; sg_icon_stat ""; sg_mask_display ""; sg_list_contents ""; sg_blockgui_xml ""
      mask help: Hardware notes: Free running counters are the least expensive in hardware. A count limited counter is implemented by combining a counter with a comparator.
      mask init: same as warplab_mimo_4x4/RSSI Clock Generator
      settings: CopyFcn=xlBlockMoveCallback(gcbh);  DeleteFcn=xlDestroyGui(gcbh);  ModelCloseFcn=xlDestroyGui(gcbh);  PreSaveFcn=xlBlockPreSaveCallback(gcbh);  PostSaveFcn=xlBlockPostSaveCallback(gcbh);  DestroyFcn=xlDestroyGui(gcbh);  OpenFcn=xlOpenGui(gcbh, 'counter_gui.xml', @counterenablement, -1)  CloseFcn=xlDestroyGui(gcbh);  MoveFcn=xlBlockMoveCallback(gcbh);
      mask Help: eval('xlWeb(xlhtmldoclink(''Counter''))');
      mask StyleString: edit,edit,popup(Free Running|Count Limited),edit,edit,popup(Up|Down|Up/Down),edit,edit,edit,popup(Signed  (2's comp)|Unsigned),edit,edit,edit,checkbox,edit,checkbox,edit,checkbox,edit,popup(on|off),edit,edit,checkbox,edit,checkbox,edit,checkbox,edit,checkbox,edit,edit,edit,edit,edit,edit,edit,edit,edit,edit
      mask Display:
      | fprintf('','COMMENT: begin icon graphics');
      | patch([0 50 50 0 ],[0 0 30 30 ],[0.77 0.82 0.91]);
      | patch([17 12 19 12 17 25 27 29 37 30 24 19 25 19 24 30 37 29 27 25 17 ],[3 8 15 22 27 27 25 27 27 20 26 21 15 9 4 10 3 3 5 3 3 ],[0.98 0.96 0.92]);
      | plot([0 0 50 50 0 ],[0 30 30 0 0 ]);
      | fprintf('','COMMENT: end icon graphics');
      | fprintf('','COMMENT: begin icon text');
      | color('black');port_label('output',1,'out');
      | fprintf('','COMMENT: end icon text');
  S-R_Latch : Subsystem
  S-R_Latch (Reverse) : Subsystem
  Scope : Scope  NumInputPorts=5
      settings: TimeRange=100000  YMin=0~-1~15469.8~0~-1  YMax=17500~1~17098.2~1~1
  WrEn : Outport
  WrAddr : Outport  Port=2
  WrAddr_zero : Outport  Port=3
  wires:
  CaptOffset/1 -> AddSub1/2
  Register/1 -> AddSub1/1, Scope/2
  AddSub1/1 -> Relational/2, Scope/3, WrAddr_zero/1
  DoneReading/1 -> S-R_Latch (Reverse)/1(S)
  Relational/1 -> S-R_Latch/1(R), Logical/1, Scope/4
  Rx Addr Counter/1 -> Scope/1, Register/1, Delay/1, Relational/1
  Start/1 -> Convert1/1
  S-R_Latch (Reverse)/1(Q) -> WrEn/1, Logical2/2
  Delay/1 -> WrAddr/1
  Convert1/1 -> Register/2, Scope/5, Logical2/1
  Logical/1 -> S-R_Latch (Reverse)/2(R)
  S-R_Latch/1(Q) -> Logical/2
  Logical2/1 -> S-R_Latch/2(S)

== system warplab_mimo_4x4/Memory Mapped I_O ==
  Constant2 : xbsIndex_r4/Constant  arith_type=Unsigned  const=0  n_bits=1  bin_pt=0  explicit_period=on  period=1  equ=P=C  opselect=C  inp2=PCIN>>17  opr=+  inp1=P  carry=CIN  dbl_ovrd=off  block_type=constant
      settings: block_version=VER_STRING_GOES_HERE
  IP2OPB_IF : Subsystem
  OPB2IP_IF : Subsystem
  Terminator : Terminator
  Terminator2 : Terminator
  ack_gen : Subsystem
  en_gen : Subsystem
  mem_if_in : Subsystem
  mem_if_out : Subsystem
  tag scope: SMWODataI_0=global, SMWODataI_1=global, SMWODataI_2=global, SMWODataI_3=global, a_valid=global, addr=global
  wires:
  OPB2IP_IF/4(OPB_DBus_Reg) -> [SMWODataI_3], [SMWODataI_2], [SMWODataI_1], [SMWODataI_0], mem_if_in/1(opb_dbus)  "opb data"
  OPB2IP_IF/1(OPB_ABus_Reg) -> en_gen/2(addr), [addr]  "opb addr"
  Constant2/1 -> IP2OPB_IF/3(SGP_retry_In), IP2OPB_IF/4(SGP_toutSup_In), IP2OPB_IF/5(SGP_errAck_In)
  mem_if_in/13(in_12_data) -> mem_if_out/15(in_12_data)
  en_gen/15(in_12_we) -> mem_if_in/14(in_12_we)
  mem_if_in/12(in_11_data) -> mem_if_out/14(in_11_data)
  en_gen/14(in_11_we) -> mem_if_in/13(in_11_we)
  mem_if_in/11(in_10_data) -> mem_if_out/13(in_10_data)
  en_gen/13(in_10_we) -> mem_if_in/12(in_10_we)
  mem_if_in/10(in_9_data) -> mem_if_out/12(in_9_data)
  en_gen/12(in_9_we) -> mem_if_in/11(in_9_we)
  mem_if_in/9(in_8_data) -> mem_if_out/11(in_8_data)
  en_gen/11(in_8_we) -> mem_if_in/10(in_8_we)
  mem_if_in/8(in_7_data) -> mem_if_out/10(in_7_data)
  en_gen/10(in_7_we) -> mem_if_in/9(in_7_we)
  mem_if_in/7(in_6_data) -> mem_if_out/9(in_6_data)
  en_gen/9(in_6_we) -> mem_if_in/8(in_6_we)
  mem_if_in/6(in_5_data) -> mem_if_out/8(in_5_data)
  en_gen/8(in_5_we) -> mem_if_in/7(in_5_we)
  mem_if_in/5(in_4_data) -> mem_if_out/7(in_4_data)
  en_gen/7(in_4_we) -> mem_if_in/6(in_4_we)
  mem_if_in/4(in_3_data) -> mem_if_out/6(in_3_data)
  en_gen/6(in_3_we) -> mem_if_in/5(in_3_we)
  mem_if_in/3(in_2_data) -> mem_if_out/5(in_2_data)
  en_gen/5(in_2_we) -> mem_if_in/4(in_2_we)
  mem_if_in/2(in_1_data) -> mem_if_out/4(in_1_data)
  en_gen/4(in_1_we) -> mem_if_in/3(in_1_we)
  mem_if_in/1(in_0_data) -> mem_if_out/3(in_0_data)
  en_gen/3(in_0_we) -> mem_if_in/2(in_0_we)
  OPB2IP_IF/3(OPB_BE_Reg) -> Terminator/1
  OPB2IP_IF/7(OPB_RNW_Reg) -> en_gen/3(rnw)  "opb read"
  OPB2IP_IF/5(OPB_seqAddr_Reg) -> Terminator2/1
  OPB2IP_IF/6(OPB_Reset) -> ack_gen/2(rst)  "opb reset"
  [ps] -> ack_gen/1(ps)  "decode"
  ack_gen/1(ack) -> en_gen/1(ack_in)
  OPB2IP_IF/2(OPB_Select_Reg) -> [a_valid]  "opb select"
  en_gen/1(ack_out) -> mem_if_out/1(ack_in)
  en_gen/2(addr_out) -> mem_if_out/2(addr)
  mem_if_out/1(sgp_DBus) -> IP2OPB_IF/1(SGP_DBus_In)
  mem_if_out/2(ack_out) -> IP2OPB_IF/2(SGP_xferAck_In)

== system warplab_mimo_4x4/Posedge ==
  D : Inport
  Delay : S-Function  LoadFcn=xlBlockLoadCallback(gcbh);  FunctionName=sysgen  Parameters=ptable_  mask(Xilinx Delay Block){infoedit=Hardware notes: A delay line is a chain, each link of which is an SRL16 followed by a flip-flop. If register retiming is enabled, the delay line is a chain of flip-flops., en_sgadvanced=, en=off, latency=1, dbl_ovrd_sgadvanced=, dbl_ovrd=off, reg_retiming_sgadvanced=, reg_retiming=off, xl_use_area_sgadvanced=, xl_use_area=off, xl_area=[0,0,0,0,0,0,0], has_advanced_control=0, sggui_pos=-1,-1,-1,-1, block_type=delay, block_version=8.2, sg_icon_stat=30,30,1,1,white,blue,0,fc531c0e, sg_mask_display=|, sg_list_contents=, sg_blockgui_xml=}
      mask sg_mask_display=|
      | fprintf('','COMMENT: begin icon graphics');
      | patch([0 30 30 0 ],[0 0 30 30 ],[0.77 0.82 0.91]);
      | patch([7 2 9 2 7 15 17 19 27 20 14 9 15 9 14 20 27 19 17 15 7 ],[3 8 15 22 27 27 25 27 27 20 26 21 15 9 4 10 3 3 5 3 3 ],[0.98 0.96 0.92]);
      | plot([0 0 30 30 0 ],[0 30 30 0 0 ]);
      | fprintf('','COMMENT: end icon graphics');
      | fprintf('','COMMENT: begin icon text');
      | color('black');disp('z^{-1}','texmode','on');
      | fprintf('','COMMENT: end icon text');
      mask prompts: infoedit ""; en_sgadvanced ""; en "Provide enable port"; dbl_ovrd_sgadvanced ""; dbl_ovrd "Override with doubles"; reg_retiming_sgadvanced ""; reg_retiming "Implement using behavioral HDL."; xl_use_area_sgadvanced ""; xl_use_area "Define FPGA area for resource estimation"; xl_area "FPGA area [slices, FFs, BRAMs, LUTs, IOBs, emb. mults, TBUFs]"; has_advanced_control ""; sggui_pos ""; block_type ""; block_version ""; sg_icon_stat ""; sg_mask_display ""; sg_list_contents ""; sg_blockgui_xml ""
      mask help: Hardware notes: A delay line is a chain, each link of which is an SRL16 followed by a flip-flop.
      mask init: same as warplab_mimo_4x4/Mem_Control/Delay
      settings: CopyFcn=xlBlockMoveCallback(gcbh);  DeleteFcn=xlDestroyGui(gcbh);  ModelCloseFcn=xlDestroyGui(gcbh);  PreSaveFcn=xlBlockPreSaveCallback(gcbh);  PostSaveFcn=xlBlockPostSaveCallback(gcbh);  DestroyFcn=xlDestroyGui(gcbh);  OpenFcn=xlOpenGui(gcbh, 'delay_gui.xml', @xlmagicenablement, -1)  CloseFcn=xlDestroyGui(gcbh);  MoveFcn=xlBlockMoveCallback(gcbh);
      mask Help: eval('xlWeb(xlhtmldoclink(''Delay''))');
      mask Display:
      | fprintf('','COMMENT: begin icon graphics');
      | patch([0 30 30 0 ],[0 0 30 30 ],[0.77 0.82 0.91]);
      | patch([7 2 9 2 7 15 17 19 27 20 14 9 15 9 14 20 27 19 17 15 7 ],[3 8 15 22 27 27 25 27 27 20 26 21 15 9 4 10 3 3 5 3 3 ],[0.98 0.96 0.92]);
      | plot([0 0 30 30 0 ],[0 30 30 0 0 ]);
      | fprintf('','COMMENT: end icon graphics');
      | fprintf('','COMMENT: begin icon text');
      | color('black');disp('z^{-1}','texmode','on');
      | fprintf('','COMMENT: end icon text');
  Inverter : S-Function  LoadFcn=xlBlockLoadCallback(gcbh);  FunctionName=sysgen  Parameters=ptable_  mask(Xilinx Inverter Block){infoedit=Bitwise logical negation (one's complement) operator., en_sgadvanced=, en=off, latency=0, dbl_ovrd_sgadvanced=, dbl_ovrd=off, xl_use_area_sgadvanced=, xl_use_area=off, xl_area=[0,0,0,0,0,0,0], has_advanced_control=0, sggui_pos=-1,-1,-1,-1, block_type=inv, block_version=8.2, sg_icon_stat=30,26,1,1,white,blue,0,1ab4a85f, sg_mask_display=|, sg_list_contents=, sg_blockgui_xml=}
      mask sg_mask_display=|
      | fprintf('','COMMENT: begin icon graphics');
      | patch([0 30 30 0 ],[0 0 26 26 ],[0.77 0.82 0.91]);
      | patch([8 4 10 4 8 15 17 19 26 20 14 10 16 10 14 20 26 19 17 15 8 ],[3 7 13 19 23 23 21 23 23 17 23 19 13 7 3 9 3 3 5 3 3 ],[0.98 0.96 0.92]);
      | plot([0 0 30 30 0 ],[0 26 26 0 0 ]);
      | fprintf('','COMMENT: end icon graphics');
      | fprintf('','COMMENT: begin icon text');
      | color('black');disp('not');
      | fprintf('','COMMENT: end icon text');
      mask prompts: infoedit ""; en_sgadvanced ""; en "Provide enable port"; dbl_ovrd_sgadvanced ""; dbl_ovrd "Override with doubles"; xl_use_area_sgadvanced ""; xl_use_area "Define FPGA area for resource estimation"; xl_area "FPGA area [slices, FFs, BRAMs, LUTs, IOBs, emb. mults, TBUFs]"; has_advanced_control ""; sggui_pos ""; block_type ""; block_version ""; sg_icon_stat ""; sg_mask_display ""; sg_list_contents ""; sg_blockgui_xml ""
      mask help: Bitwise logical negation (one's complement) operator.
      mask init: same as warplab_mimo_4x4/Inverter
      settings: CopyFcn=xlBlockMoveCallback(gcbh);  DeleteFcn=xlDestroyGui(gcbh);  ModelCloseFcn=xlDestroyGui(gcbh);  PreSaveFcn=xlBlockPreSaveCallback(gcbh);  PostSaveFcn=xlBlockPostSaveCallback(gcbh);  DestroyFcn=xlDestroyGui(gcbh);  OpenFcn=xlOpenGui(gcbh, 'inv_gui.xml', @xlmagicenablement, -1)  CloseFcn=xlDestroyGui(gcbh);  MoveFcn=xlBlockMoveCallback(gcbh);
      mask Help: eval('xlWeb(xlhtmldoclink(''Inverter''))');
      mask Display:
      | fprintf('','COMMENT: begin icon graphics');
      | patch([0 30 30 0 ],[0 0 26 26 ],[0.77 0.82 0.91]);
      | patch([8 4 10 4 8 15 17 19 26 20 14 10 16 10 14 20 26 19 17 15 8 ],[3 7 13 19 23 23 21 23 23 17 23 19 13 7 3 9 3 3 5 3 3 ],[0.98 0.96 0.92]);
      | plot([0 0 30 30 0 ],[0 26 26 0 0 ]);
      | fprintf('','COMMENT: end icon graphics');
      | fprintf('','COMMENT: begin icon text');
      | color('black');disp('not');
      | fprintf('','COMMENT: end icon text');
  Logical : S-Function  LoadFcn=xlBlockLoadCallback(gcbh);  FunctionName=sysgen  Parameters=ptable_  mask(Xilinx Logical Block Block){logical_function_sgadvanced=, logical_function=AND, inputs=2, en_sgadvanced=, en=off, latency=0, precision_sgadvanced=, precision=Full, arith_type_sgadvanced=, arith_type=Unsigned, n_bits=16, bin_pt=0, align_bp_sgadvanced=, align_bp=on, dbl_ovrd_sgadvanced=, dbl_ovrd=off, xl_use_area_sgadvanced=, xl_use_area=off, xl_area=[0,0,0,0,0,0,0], overflow=, quantization=, has_advanced_control=0, sggui_pos=-1,-1,-1,-1, block_type=logical, block_version=8.2, sg_icon_stat=35,42,2,1,white,blue,0,087b5522, sg_mask_display=|, sg_list_contents=, sg_blockgui_xml=}
      mask sg_mask_display=|
      | fprintf('','COMMENT: begin icon graphics');
      | patch([0 35 35 0 ],[0 0 42 42 ],[0.77 0.82 0.91]);
      | patch([8 2 10 2 8 17 20 23 33 25 18 13 21 13 18 25 33 23 20 17 8 ],[7 13 21 29 35 35 32 35 35 27 34 29 21 13 8 15 7 7 10 7 7 ],[0.98 0.96 0.92]);
      | plot([0 0 35 35 0 ],[0 42 42 0 0 ]);
      | fprintf('','COMMENT: end icon graphics');
      | fprintf('','COMMENT: begin icon text');
      | color('black');disp('\newlineand\newlinez^{-0}','texmode','on');
      | fprintf('','COMMENT: end icon text');
      mask prompts: logical_function_sgadvanced ""; logical_function "Logical function"; inputs "Number of inputs"; en_sgadvanced ""; en "Provide enable port"; precision_sgadvanced ""; arith_type_sgadvanced ""; arith_type "Output Type"; n_bits "Number of bits"; bin_pt "Binary point"; align_bp_sgadvanced ""; align_bp "Align binary point"; dbl_ovrd_sgadvanced ""; dbl_ovrd "Override with doubles"; xl_use_area_sgadvanced ""; xl_use_area "Define FPGA area for resource estimation"; xl_area "FPGA area [slices, FFs, BRAMs, LUTs, IOBs, emb. mults, TBUFs]"; overflow ""; quantization ""; has_advanced_control ""; sggui_pos ""; block_type ""; block_version ""; sg_icon_stat ""; sg_mask_display ""; sg_list_contents ""; sg_blockgui_xml ""
      mask help: Xilinx Logical Block
      mask init: same as warplab_mimo_4x4/Logical
      settings: CopyFcn=xlBlockMoveCallback(gcbh);  DeleteFcn=xlDestroyGui(gcbh);  ModelCloseFcn=xlDestroyGui(gcbh);  PreSaveFcn=xlBlockPreSaveCallback(gcbh);  PostSaveFcn=xlBlockPostSaveCallback(gcbh);  DestroyFcn=xlDestroyGui(gcbh);  OpenFcn=xlOpenGui(gcbh, 'logical_gui.xml', @logicalenablement, -1)  CloseFcn=xlDestroyGui(gcbh);  MoveFcn=xlBlockMoveCallback(gcbh);
      mask Help: eval('xlWeb(xlhtmldoclink(''Logical''))');
      mask StyleString: edit,popup(AND|NAND|OR|NOR|XOR|XNOR),edit,edit,checkbox,edit,edit,popup(Full|User Defined),edit,popup(Signed  (2's comp)|Unsigned),edit,edit,edit,checkbox,edit,checkbox,edit,checkbox,edit,edit,edit,edit,edit,edit,edit,edit,edit,edit,edit
      mask Display:
      | fprintf('','COMMENT: begin icon graphics');
      | patch([0 35 35 0 ],[0 0 42 42 ],[0.77 0.82 0.91]);
      | patch([8 2 10 2 8 17 20 23 33 25 18 13 21 13 18 25 33 23 20 17 8 ],[7 13 21 29 35 35 32 35 35 27 34 29 21 13 8 15 7 7 10 7 7 ],[0.98 0.96 0.92]);
      | plot([0 0 35 35 0 ],[0 42 42 0 0 ]);
      | fprintf('','COMMENT: end icon graphics');
      | fprintf('','COMMENT: begin icon text');
      | color('black');disp('\newlineand\newlinez^{-0}','texmode','on');
      | fprintf('','COMMENT: end icon text');
  Q : Outport
  wires:
  D/1 -> Inverter/1, Logical/1
  Inverter/1 -> Delay/1
  Delay/1 -> Logical/2
  Logical/1 -> Q/1
